simulink model "spring_mass_damper"  (R2025b)
settings: Solver=VariableStepAuto  StartTime=0.0  StopTime=10.0  RelTol=1e-3
model workspace (MAT data in the model file):
  m = 0
settings Model: Creator=Junch  LastModifiedBy=Junch

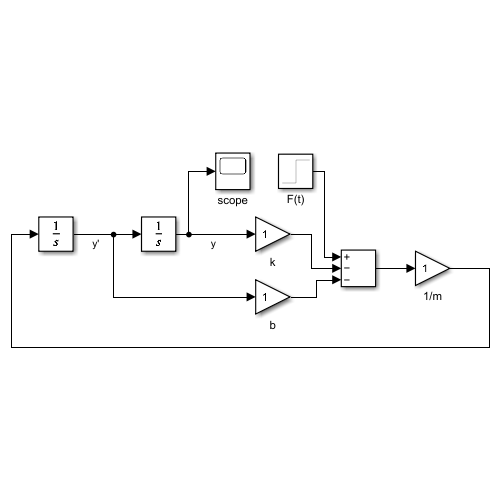
[thumbnail: Simulink's stored preview of the top-level diagram]
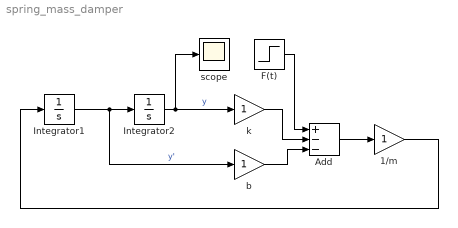
== system spring_mass_damper ==
  1/m : Gain
  Add : Sum  Inputs=+--
  F(t) : Step  SampleTime=0
  Integrator1 : Integrator
  Integrator2 : Integrator
  b : Gain
  k : Gain
  scope : Scope
      settings: ActiveDisplayYMinimum=-0.1453713652748744  ActiveDisplayYMaximum=1.30834228747387
  wires:
  Integrator1/1 -> b/1, Integrator2/1  "y'"
  Integrator2/1 -> k/1, scope/1  "y"
  k/1 -> Add/2
  b/1 -> Add/3
  F(t)/1 -> Add/1
  Add/1 -> 1/m/1
  1/m/1 -> Integrator1/1
